simulink model "SynchGenerator_breaker_cst_W_load_Increased"  (Simulink 7.6)
settings: Solver=ode23tb  StartTime=0.0  StopTime=3  RelTol=1e-3
libraries: powerlib x10
settings Model: Creator=kif  LastModifiedBy=kif

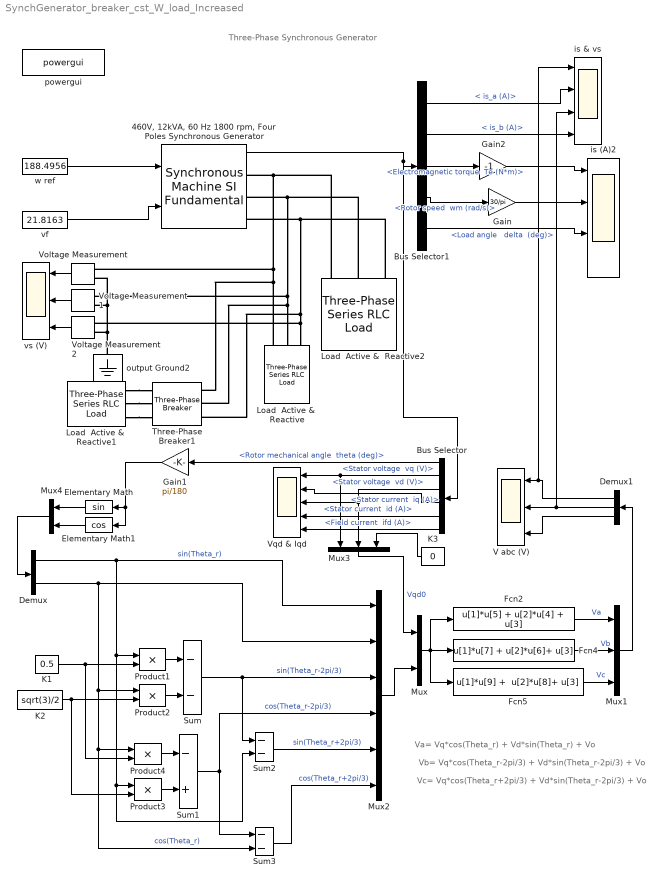
== system SynchGenerator_breaker_cst_W_load_Increased ==
  note: Three-Phase Synchronous Generator
  note: Va= Vq*cos(Theta_r) + Vd*sin(Theta_r) + Vo
  note: Vc= Vq*cos(Theta_r+2pi/3) + Vd*sin(Theta_r-2pi/3) + Vo
  note: Vb= Vq*cos(Theta_r-2pi/3) + Vd*sin(Theta_r-2pi/3) + Vo
  "460V, 12kVA, 60 Hz 1800 rpm, Four Poles Synchronous Generator" : powerlib/Machines/Synchronous Machine SI Fundamental  DialogController=POWERSYS.PowerSysDialog  SystemSampleTime=-1  PresetModel=No  MechanicalLoad=Speed w  ShowDetailedParameters=on  RotorType=Salient-pole  NominalParameters="[ 11.9e3 460  60  0]"  Stator=[ .26 1.14e-3 13.7e-3 11.0e-3 ]  Field=[ 0.3 2.1e-3 ]  Dampers2=[ 1 2 3 4 5 6 ]  Dampers1=[ 0.0224 1.4e-3 0.02 1e-3 ]  Mechanical=[ 24.9 0 2]  PolePairs=2  InitialConditions=[0 -111.483 0 0 0 -173.297 66.7033 -53.2967 17.88]  SetSaturation=off  Saturation=[46.376,51.647,61.167,66.773,72.147,78.393,86.24,95.347,105.58;644,708.2,816.2,870.87,917.13,962.47,1012,1059.3,1104.5]  DisplayVfd=off  Units=SI fundamental parameters  LoadFlowParameters=[1 -50000 0 0 0]  TsPowergui=0  TsBlock=-1  IterativeModel=Forward Euler
      link override From: GotoTag=tp5344ed80_c545_43ed_8e4c_276f4009b387
      settings: AttributesFormatString=\n
  Bus Selector : BusSelector  OutputSignals="Mechanical.Rotor mechanical angle  theta (deg),dq0 components.Stator voltage  vq (V),dq0 components.Stator voltage  vd (V),dq0 components.Stator current  iq (A),dq0 components.Stator current  id (A),dq0 components.Field current  ifd (A)"
  Bus Selector1 : BusSelector  OutputSignals="Stator current. is_a (A),Stator current. is_b (A),Mechanical.Electromagnetic torque  Te (N*m),Mechanical.Rotor speed  wm (rad/s),Load angle   delta  (deg)"
  Demux : Demux  Outputs=2
  Demux1 : Demux  Outputs=3
  Elementary Math : Trigonometry
  Elementary Math1 : Trigonometry  Operator=cos
  Fcn2 : Fcn  Expr=u[1]*u[5] + u[2]*u[4] + u[3]
  Fcn4 : Fcn  Expr="u[1]*u[7] +  u[2]*u[6]+ u[3]"
  Fcn5 : Fcn  Expr="u[1]*u[9] +  u[2]*u[8]+ u[3]"
  Gain : Gain  Gain=30/pi  SaturateOnIntegerOverflow=on  OutDataTypeStr=Inherit: Same as input  ParamDataTypeStr=Inherit: Same as input
  Gain1 : Gain  Gain=pi/180  SaturateOnIntegerOverflow=on  OutDataTypeStr=Inherit: Same as input  ParamDataTypeStr=Inherit: Same as input
  Gain2 : Gain  Gain=-1  SaturateOnIntegerOverflow=on  OutDataTypeStr=Inherit: Same as input  ParamDataTypeStr=Inherit: Same as input
  K1 : Constant  Value=0.5
  K2 : Constant  Value=sqrt(3)/2
  K3 : Constant  Value=0
  Load  Active &  Reactive : powerlib/Elements/Three-Phase Series RLC Load  DialogController=POWERSYS.PowerSysDialog  PhysicalDomain=powersysdomain  SubClassName=unknown  LeftPortType=p1  RightPortType=p1  LConnTagsString=A|B|C  Configuration=Y (grounded)  NominalVoltage=460  NominalFrequency=60  ActivePower=1000  InductivePower=100  CapacitivePower=0  Measurements=None
  Load  Active &  Reactive1 : powerlib/Elements/Three-Phase Series RLC Load  DialogController=POWERSYS.PowerSysDialog  PhysicalDomain=powersysdomain  SubClassName=unknown  LeftPortType=p1  RightPortType=p1  LConnTagsString=A|B|C  Configuration=Y (grounded)  NominalVoltage=460  NominalFrequency=60  ActivePower=10000  InductivePower=1000  CapacitivePower=0  Measurements=None
  Load  Active &  Reactive2 : powerlib/Elements/Three-Phase Series RLC Load  DialogController=POWERSYS.PowerSysDialog  PhysicalDomain=powersysdomain  SubClassName=unknown  LeftPortType=p1  RightPortType=p1  LConnTagsString=A|B|C  Configuration=Y (grounded)  NominalVoltage=460  NominalFrequency=60  ActivePower=100  InductivePower=0  CapacitivePower=0  Measurements=None
  Mux : Mux  Inputs=2
  Mux1 : Mux  Inputs=3
  Mux2 : Mux  Inputs=6
  Mux3 : Mux  Inputs=3
  Mux4 : Mux  Inputs=2
  Product{1..4} (4 alike) : Product  SaturateOnIntegerOverflow=on  InputSameDT=on  OutDataTypeStr=Inherit: Same as first input
  Sum : Sum  Inputs=--  SaturateOnIntegerOverflow=on  InputSameDT=on  OutDataTypeStr=Inherit: Same as first input
  Sum1 : Sum  Inputs=-+  SaturateOnIntegerOverflow=on  InputSameDT=on  OutDataTypeStr=Inherit: Same as first input
  Sum2 : Sum  Inputs=--  SaturateOnIntegerOverflow=on  InputSameDT=on  OutDataTypeStr=Inherit: Same as first input
  Sum3 : Sum  Inputs=--  SaturateOnIntegerOverflow=on  InputSameDT=on  OutDataTypeStr=Inherit: Same as first input
  Three-Phase Breaker1 : powerlib/Elements/Three-Phase Breaker  DialogController=POWERSYS.PowerSysDialog  SystemSampleTime=-1  InitialState=open  SwitchA=on  SwitchB=on  SwitchC=on  SwitchTimes=[1.5]  External=off  BreakerResistance=0.001  SnubberResistance=1e6  SnubberCapacitance=inf  Measurements=None
  V abc (V) : Scope  NumInputPorts=3
      settings: YMin=-3.5~-5~-5  YMax=3.5~5~5  DataFormat=Structure
  Voltage Measurement : powerlib/Measurements/Voltage Measurement  DialogController=POWERSYS.PowerSysDialog  SystemSampleTime=-1  PhasorSimulation=off  OutputType=Complex  PSBequivalent=0
  Voltage Measurement1 : powerlib/Measurements/Voltage Measurement  DialogController=POWERSYS.PowerSysDialog  SystemSampleTime=-1  PhasorSimulation=off  OutputType=Complex  PSBequivalent=0
  Voltage Measurement2 : powerlib/Measurements/Voltage Measurement  DialogController=POWERSYS.PowerSysDialog  SystemSampleTime=-1  PhasorSimulation=off  OutputType=Complex  PSBequivalent=0
  Vqd & Iqd : Scope  NumInputPorts=5
      settings: YMin=-3.5~-5~-5~-5~-5  YMax=3.5~5~5~5~5  SaveName=ScopeData4  DataFormat=Structure
  is & vs : Scope  NumInputPorts=4
      settings: YMin=-300~-75~-300~-75  YMax=300~75~300~75  SaveName=ScopeData2  DataFormat=Structure
  is (A)2 : Scope  NumInputPorts=4
      settings: TimeRange=4  YMin=-600~1795~-40~-10  YMax=400~1815~60~300  SaveName=ScopeData3  DataFormat=Structure
  output Ground2 : powerlib/Elements/Ground  DialogController=POWERSYS.PowerSysDialog  PhysicalDomain=powersysdomain  SubClassName=unknown  LeftPortType=p1  RightPortType=p1  LConnTagsString=a
  powergui : powerlib/powergui  Priority=2  SystemSampleTime=-1  SimulationMode=Continuous  SampleTime=1  frequency=60  SPID=off  DisableSnubberDevices=off  DisableRonSwitches=off  DisableVfSwitches=off  SwTol=0  Interpol=off  frequencyindice=60  echomessages=off  HookPort=off  DisplayEquations=off  FunctionMessages=off  EnableUseOfTLC=off  x0status=blocks  RestoreLinks=warning  ResistiveCurrentMeasurement=off  Frange=logspace(0,3,50)  Ylog=off  Xlog=off  ShowGrid=off  save=off  variable=ZData  ZoomFFT=on  StartTime=0.0  cycles=2  DisplayStyle=off  fundamental=60  FreqAxis=off  MaxFrequency=1000  frequencyindicesteady=1  RmsSteady=1  display=off  Ts=0  methode=off
  vf : Constant  Value=21.8163
  vs (V) : Scope  NumInputPorts=3
      settings: YMin=-500~-400~-450  YMax=400~400~400  DataFormat=Structure
  w ref : Constant  Value=188.4956
  wires:
  vf/1 -> "460V, 12kVA, 60 Hz 1800 rpm, Four Poles Synchronous Generator"/2
  Voltage Measurement/1 -> vs (V)/1
  Voltage Measurement1/1 -> vs (V)/2
  Voltage Measurement2/1 -> vs (V)/3
  Fcn5/1 -> Mux1/3  "Vc"
  Fcn2/1 -> Mux1/1  "Va"
  Mux1/1 -> Demux1/1
  Mux/1 -> Fcn2/1, Fcn5/1, Fcn4/1
  Sum1/1 -> Sum3/1, Mux2/4  "cos(Theta_r-2pi/3)"
  Sum/1 -> Sum2/1, Mux2/3  "sin(Theta_r-2pi/3)"
  K2/1 -> Product3/2, Product2/2
  K1/1 -> Product4/2, Product1/2
  Sum2/1 -> Mux2/5  "sin(Theta_r+2pi/3)"
  Sum3/1 -> Mux2/6  "cos(Theta_r+2pi/3)"
  Product3/1 -> Sum1/2
  Product4/1 -> Sum1/1
  Product2/1 -> Sum/2
  Product1/1 -> Sum/1
  Demux/1 -> Mux2/1, Sum2/2, Product3/1, Product1/1  "sin(Theta_r)"
  Demux/2 -> Mux2/2, Product2/1, Product4/1, Sum3/2  "cos(Theta_r)"
  Mux4/1 -> Demux/1
  Mux2/1 -> Mux/2
  Mux3/1 -> Mux/1  "Vqd0"
  Elementary Math/1 -> Mux4/1
  Elementary Math1/1 -> Mux4/2
  Demux1/1 -> V abc (V)/1, is & vs/1
  Demux1/2 -> V abc (V)/2, is & vs/3
  Demux1/3 -> V abc (V)/3
  Bus Selector/2 -> Mux3/1, Vqd & Iqd/1  "<Stator voltage  vq (V)>"
  Bus Selector/3 -> Mux3/2, Vqd & Iqd/3  "<Stator voltage  vd (V)>"
  K3/1 -> Mux3/3
  Bus Selector/1 -> Gain1/1  "<Rotor mechanical angle  theta (deg)>"
  Fcn4/1 -> Mux1/2  "Vb"
  Bus Selector1/1 -> is & vs/2  "< is_a (A)>"
  Bus Selector1/2 -> is & vs/4  "< is_b (A)>"
  Bus Selector1/3 -> Gain2/1  "<Electromagnetic torque  Te (N*m)>"
  Bus Selector1/4 -> Gain/1  "<Rotor speed  wm (rad/s)>"
  Bus Selector1/5 -> is (A)2/3  "<Load angle   delta  (deg)>"
  "460V, 12kVA, 60 Hz 1800 rpm, Four Poles Synchronous Generator"/1 -> Bus Selector1/1, Bus Selector/1
  Gain/1 -> is (A)2/2
  Gain1/1 -> Elementary Math/1, Elementary Math1/1
  Bus Selector/5 -> Vqd & Iqd/4  "<Stator current  id (A)>"
  Bus Selector/4 -> Vqd & Iqd/2  "<Stator current  iq (A)>"
  Bus Selector/6 -> Vqd & Iqd/5  "<Field current  ifd (A)>"
  w ref/1 -> "460V, 12kVA, 60 Hz 1800 rpm, Four Poles Synchronous Generator"/1
  Gain2/1 -> is (A)2/1
  connections:
  Load  Active &  Reactive2/LConn1 -- Load  Active &  Reactive/LConn1 -- Three-Phase Breaker1/LConn1 -- Voltage Measurement/LConn1 -- "460V, 12kVA, 60 Hz 1800 rpm, Four Poles Synchronous Generator"/RConn1
  Load  Active &  Reactive2/LConn2 -- Load  Active &  Reactive/LConn2 -- Three-Phase Breaker1/LConn2 -- Voltage Measurement1/LConn1 -- "460V, 12kVA, 60 Hz 1800 rpm, Four Poles Synchronous Generator"/RConn2
  Load  Active &  Reactive2/LConn3 -- Load  Active &  Reactive/LConn3 -- Voltage Measurement2/LConn1 -- Three-Phase Breaker1/LConn3 -- "460V, 12kVA, 60 Hz 1800 rpm, Four Poles Synchronous Generator"/RConn3
  Load  Active &  Reactive1/LConn2 -- Three-Phase Breaker1/RConn2
  Load  Active &  Reactive1/LConn1 -- Three-Phase Breaker1/RConn1
  Load  Active &  Reactive1/LConn3 -- Three-Phase Breaker1/RConn3
  output Ground2/LConn1 -- Voltage Measurement/LConn2 -- Voltage Measurement1/LConn2 -- Voltage Measurement2/LConn2
